simulink model "filtration0510"  (R2024a)
settings: Solver=VariableStepAuto  StartTime=0.0  StopTime=100  RelTol=1e-3
libraries: dspfdesign x3, simulink x1, dspstat3 x1
settings Model: Creator=pupkinzalupkin  LastModifiedBy=pupkinzalupkin

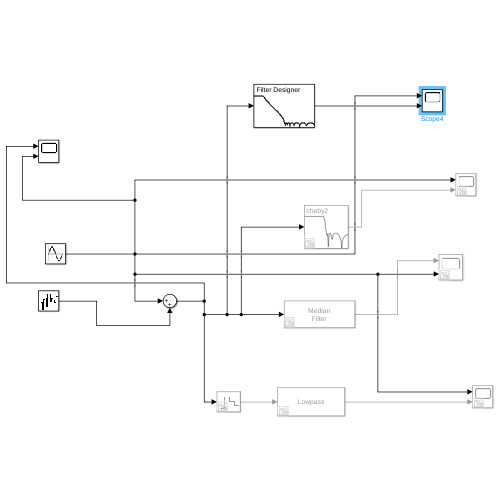
[thumbnail: Simulink's stored preview of the top-level diagram]
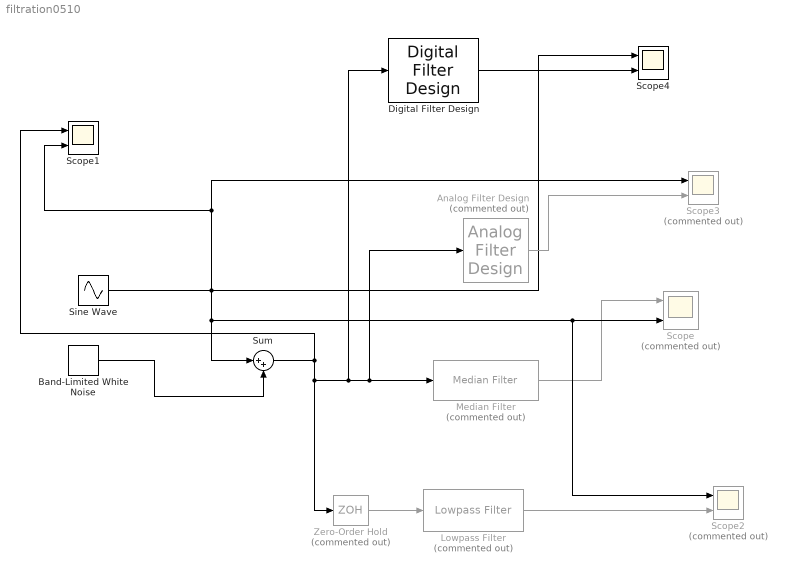
== system filtration0510 ==
  Analog Filter Design : dspfdesign/Analog Filter Design  Commented=on  method=Chebyshev II  filttype=Lowpass  N=8  Wlo=1.6  Whi=80  Rp=2  Rs=40
  Band-Limited White Noise : simulink/Sources/Band-Limited White Noise  Cov=[0.1]  Ts=0.2  seed=[2334]
  Digital Filter Design : dspfdesign/Digital Filter Design  mwdsp_browser_bugfix_var=off
  Lowpass Filter : dspfdesign/Lowpass Filter  Commented=on  FilterType=FIR  DesignForMinimumOrder=on  FilterOrder=50  PassbandFrequency=1e3  StopbandFrequency=3e3  PassbandRipple=0.9  StopbandAttenuation=150  SampleRateMode=Specify on dialog  SampleRate=24000  SimulateUsing=Interpreted execution  roundingMode=Floor  coeffsDataTypeStr=fixdt(1,16)
  Median Filter : dspstat3/Median Filter  Commented=on  WindowLength=10  SimulateUsing=Interpreted execution
      settings: LibrarySourceBlock=|
      | dspfdesign/Median
      | Filter
  Scope : Scope  Commented=on  NumInputPorts=2
  Scope1 : Scope  NumInputPorts=2
  Scope2 : Scope  Commented=on  NumInputPorts=2
  Scope3 : Scope  Commented=on  NumInputPorts=2
  Scope4 : Scope  NumInputPorts=2
  Sine Wave : Sin  SampleTime=0
  Sum : Sum  Inputs=|++
  Zero-Order Hold : ZeroOrderHold  Commented=on  SampleTime=-1
  wires:
  Band-Limited White Noise/1 -> Sum/2
  Sum/1 -> Scope1/1, Digital Filter Design/1, Analog Filter Design/1, Median Filter/1, Zero-Order Hold/1
  Median Filter/1 -> Scope/1
  Sine Wave/1 -> Scope4/1, Scope2/1, Scope/2, Sum/1, Scope3/1, Scope1/2
  Lowpass Filter/1 -> Scope2/2
  Zero-Order Hold/1 -> Lowpass Filter/1
  Analog Filter Design/1 -> Scope3/2
  Digital Filter Design/1 -> Scope4/2
